simulink model "sensor_readout_frontend"  (R2022a)
settings: Solver=ode45  StartTime=0.0  StopTime=12  RelTol=1e-6  AbsTol=1e-8
settings Model: Creator=HJL  LastModifiedBy=HJL

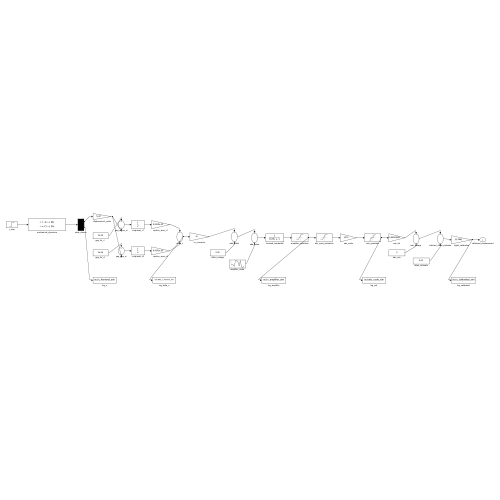
[thumbnail: Simulink's stored preview of the top-level diagram]
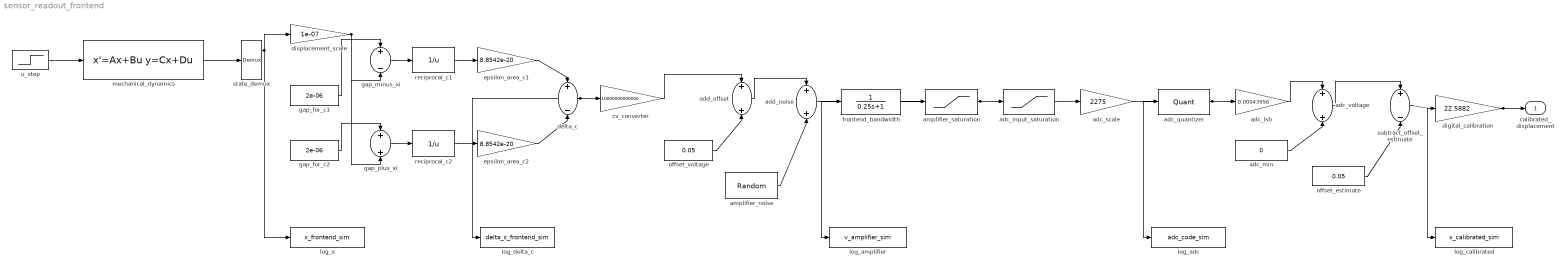
== system sensor_readout_frontend ==
  adc_input_saturation : Saturate  UpperLimit=1.8  LowerLimit=0
  adc_lsb : Gain  Gain=0.00043956
  adc_min : Constant  Value=0
  adc_quantizer : Quantizer  QuantizationInterval=1
  adc_scale : Gain  Gain=2275
  adc_voltage : Sum
  add_noise : Sum
  add_offset : Sum
  amplifier_noise : RandomNumber  Variance=2.5e-07  Seed=23  SampleTime=0.01
  amplifier_saturation : Saturate  UpperLimit=1.8  LowerLimit=0
  cv_converter : Gain  Gain=10000000000000
  delta_c : Sum  Inputs=+-
  digital_calibration : Gain  Gain=22.5882
  displacement_scale : Gain  Gain=1e-07
  epsilon_area_c1 : Gain  Gain=8.8542e-20
  epsilon_area_c2 : Gain  Gain=8.8542e-20
  frontend_bandwidth : TransferFcn  Denominator=[0.25 1]
  gap_for_c1 : Constant  Value=2e-06
  gap_for_c2 : Constant  Value=2e-06
  gap_minus_xi : Sum  Inputs=+-
  gap_plus_xi : Sum
  log_adc : ToWorkspace  VariableName=adc_code_sim  SaveFormat=Timeseries  SampleTime=-1
  log_amplifier : ToWorkspace  VariableName=v_amplifier_sim  SaveFormat=Timeseries  SampleTime=-1
  log_calibrated : ToWorkspace  VariableName=x_calibrated_sim  SaveFormat=Timeseries  SampleTime=-1
  log_delta_c : ToWorkspace  VariableName=delta_c_frontend_sim  SaveFormat=Timeseries  SampleTime=-1
  log_x : ToWorkspace  VariableName=x_frontend_sim  SaveFormat=Timeseries  SampleTime=-1
  mechanical_dynamics : StateSpace  A=[0 1; -1.2 -0.2]  B=[0; 1]  C=[1 0; 0 1]  D=[0; 0]  InitialCondition=[0; 0]
  offset_estimate : Constant  Value=0.05
  offset_voltage : Constant  Value=0.05
  reciprocal_c1 : Math  Operator=reciprocal
  reciprocal_c2 : Math  Operator=reciprocal
  state_demux : Demux  Outputs=2
  subtract_offset_estimate : Sum  Inputs=+-
  u_step : Step  SampleTime=0
  calibrated_displacement : Outport
  wires:
  u_step/1 -> mechanical_dynamics/1
  mechanical_dynamics/1 -> state_demux/1
  state_demux/1 -> displacement_scale/1, log_x/1
  displacement_scale/1 -> gap_minus_xi/2, gap_plus_xi/2
  gap_for_c1/1 -> gap_minus_xi/1
  gap_for_c2/1 -> gap_plus_xi/1
  gap_minus_xi/1 -> reciprocal_c1/1
  gap_plus_xi/1 -> reciprocal_c2/1
  reciprocal_c1/1 -> epsilon_area_c1/1
  reciprocal_c2/1 -> epsilon_area_c2/1
  epsilon_area_c1/1 -> delta_c/1
  epsilon_area_c2/1 -> delta_c/2
  delta_c/1 -> cv_converter/1, log_delta_c/1
  cv_converter/1 -> add_offset/1
  offset_voltage/1 -> add_offset/2
  add_offset/1 -> add_noise/1
  amplifier_noise/1 -> add_noise/2
  add_noise/1 -> frontend_bandwidth/1
  frontend_bandwidth/1 -> amplifier_saturation/1
  amplifier_saturation/1 -> adc_input_saturation/1, log_amplifier/1
  adc_input_saturation/1 -> adc_scale/1
  adc_scale/1 -> adc_quantizer/1
  adc_quantizer/1 -> adc_lsb/1, log_adc/1
  adc_lsb/1 -> adc_voltage/1
  adc_min/1 -> adc_voltage/2
  adc_voltage/1 -> subtract_offset_estimate/1
  offset_estimate/1 -> subtract_offset_estimate/2
  subtract_offset_estimate/1 -> digital_calibration/1
  digital_calibration/1 -> calibrated_displacement/1, log_calibrated/1
